simulink model "debugUDP"  (Simulink 7.2)
settings: Solver=ode1  SolverMode=SingleTasking  StartTime=0  StopTime=FAKEExpData.t(end)+4  FixedStep=0.001  RelTol=1e-3
PreLoadFcn:
  | InitModel
  | make
InitFcn:
  | InitModel
  | make
values from neighbouring files (symbols this model uses):
  D = SSD.D    [Ext_MPCPara.m]
  Ts = 0.002    [DSC_Control_Analysis.m]    (also in DSC_Control_Analysis_Exp.m; DSC_Speed_Control_Analysis.m; EC_params_nissan.m; Ext_MPCPara.m = SSD.Ts)
undefined symbols (not defined in the file or in its folder): FAKEExpData
libraries: xpclib x7, simulink x3
settings Model: Creator=cgadda  LastModifiedBy=ddl  ExtModeArmWhenConnect=off  ExtModeAutoUpdateStatusClock=off  BufferReuse=off
settings DataIOCC: LimitDataPoints=off  TimeSaveName=t  OutputSaveName=y  SignalLoggingName=sigsOut
settings OptimizationCC: BlockReduction=off  BooleanDataType=off  OptimizeBlockIOStorage=off  BufferReuse=off  EnforceIntegerDowncast=off  ExpressionFolding=off  FoldNonRolledExpr=off  LocalBlockOutputs=off  InitFltsAndDblsToZero=on
settings DebuggingCC: SaveWithParameterizedLinksMsg=none  SolverPrmCheckMsg=none  MultiTaskDSMMsg=warning  MultiTaskCondExecSysMsg=none
settings HardwareCC: ProdIntDivRoundTo=Zero  ProdEndianess=LittleEndian  ProdHWDeviceType=Generic->32-bit x86 compatible  TargetIntDivRoundTo=Zero  TargetEndianess=LittleEndian  TargetHWDeviceType=32-bit xPC Target (Intel Pentium)
settings RTWCC: SystemTargetFile=xpctarget.tlc  TemplateMakefile=xpc_default_tmf  Description=xPC Target  ProcessScript=xpctarget_make_rtw_hook  IncludeERTFirstTime=on  RTWCompilerOptimization=On
settings xpcTargetCC: TargetFcnLib=ansi_tfl_tmw.mat  TargetFunctionLibrary=ANSI_C  PortableWordSizes=off  RL32LogBufSizeModifier=25000000  xPCisDownloadable=off

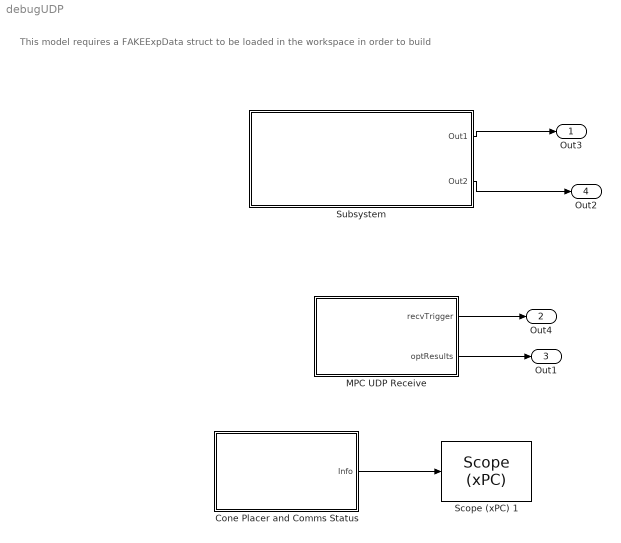
== system debugUDP ==
  note: This model requires a FAKEExpData struct
      | to be loaded in the workspace in order
      | to build
  Cone Placer and Comms Status : Subsystem
  MPC UDP Receive : Subsystem
  Scope (xPC) 1 : xpclib/Misc./Scope (xPC)   SystemSampleTime=-1  scopeno=1  scopetype=Target  autostart=on  viewmode=Numerical  formatstr="' Bumper E Pos [m]:    %4.2f, Bumper N Pos [m]:    %4.2f, Num Laptop Msgs: %5.0f, Num Veh Msgs:    %5.0f'"  grid=on  ylimits=[0,0]  nosamples=round(1/Ts)  noprepostsamples=0  interleave=1  triggermode=FreeRun  triggersignal=1  triggerlevel=0.0  triggerslope=Either  triggerscope=1  triggersample=0  filename=data.dat  mode=Lazy  writesize=512  autorestart=off
  Subsystem : Subsystem
  Out3 : Outport  OutDataType=sfix(16)  OutScaling=2^0
  Out4 : Outport  Port=2  OutDataType=sfix(16)  OutScaling=2^0
  Out1 : Outport  Port=3  OutDataType=sfix(16)  OutScaling=2^0
  Out2 : Outport  Port=4  OutDataType=sfix(16)  OutScaling=2^0
  wires:
  Subsystem/2(Out2) -> Out2/1
  MPC UDP Receive/2(optResults) -> Out1/1
  MPC UDP Receive/1(recvTrigger) -> Out4/1
  Subsystem/1(Out1) -> Out3/1
  Cone Placer and Comms Status/1(Info) -> Scope (xPC) 1/1

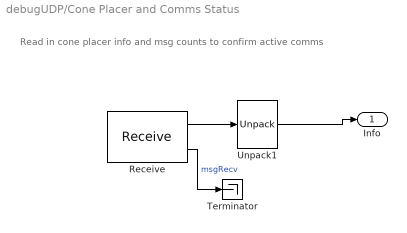
== system debugUDP/Cone Placer and Comms Status ==
  note: Read in cone
      | placer info and
      | msg counts to confirm
      | active comms
  Receive : xpclib/UDP/Receive  ipAddress=171.64.164.232  ipPort=25012  width=4*8  sampletime=-1
  Terminator : Terminator
  Unpack1 : xpclib/UDP/Unpack  dimensions={4}  datatypes={'double'}  byteAlign=1
  Info : Outport  OutDataType=sfix(16)  OutScaling=2^0
  wires:
  Receive/1 -> Unpack1/1
  Unpack1/1 -> Info/1
  Receive/2 -> Terminator/1  "msgRecv"

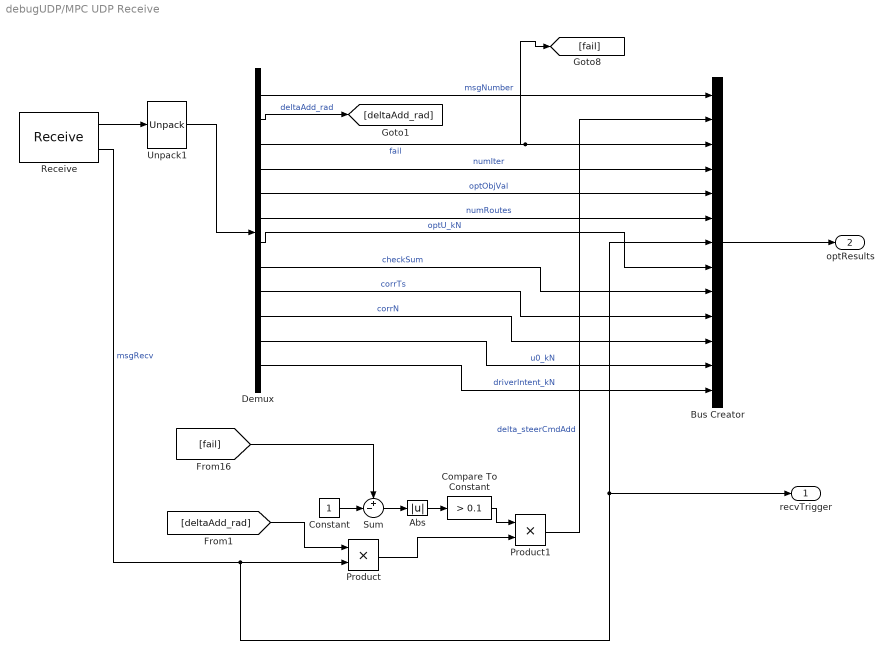
== system debugUDP/MPC UDP Receive ==
  Abs : Abs  OutDataType=sfix(16)  OutScaling=2^0
  Bus Creator : BusCreator  Inputs=13
  Compare To Constant : simulink/Logic and Bit Operations/Compare To Constant  SystemSampleTime=-1  relop=>  const=0.1  LogicOutDataTypeMode=uint8  ZeroCross=off
  Constant : Constant  OutDataType=sfix(16)  OutScaling=2^0
  Demux : Demux  Outputs=12
  Product : Product  OutDataType=sfix(16)  OutScaling=2^0  RndMeth=Zero
  Product1 : Product  OutDataType=sfix(16)  OutScaling=2^0  RndMeth=Zero
  Receive : xpclib/UDP/Receive  ipAddress=171.64.164.232  ipPort=25011  width=12*8  sampletime=-1
  Sum : Sum  Inputs=+-|  OutDataType=sfix(16)  OutScaling=2^0
  Unpack1 : xpclib/UDP/Unpack  dimensions={12}  datatypes={'double'}  byteAlign=1
  recvTrigger : Outport  OutDataType=sfix(16)  OutScaling=2^0
  optResults : Outport  Port=2  OutDataType=sfix(16)  OutScaling=2^0
  wires:
  Receive/1 -> Unpack1/1
  Receive/2 -> Product/2, Bus Creator/7, recvTrigger/1  "msgRecv"
  Unpack1/1 -> Demux/1
  Demux/1 -> Bus Creator/1  "msgNumber"
  Demux/3 -> Bus Creator/3, [fail]  "fail"
  Demux/4 -> Bus Creator/4  "numIter"
  Demux/5 -> Bus Creator/5  "optObjVal"
  Product1/1 -> Bus Creator/2  "delta_steerCmdAdd"
  Constant/1 -> Sum/2
  Sum/1 -> Abs/1
  Abs/1 -> Compare To Constant/1
  Compare To Constant/1 -> Product1/1
  Product/1 -> Product1/2
  Bus Creator/1 -> optResults/1
  Demux/7 -> Bus Creator/8  "optU_kN"
  Demux/8 -> Bus Creator/9  "checkSum"
  Demux/9 -> Bus Creator/10  "corrTs"
  Demux/10 -> Bus Creator/11  "corrN"
  Demux/11 -> Bus Creator/12  "u0_kN"
  Demux/12 -> Bus Creator/13  "driverIntent_kN"
  [fail] -> Sum/1
  Demux/2 -> [deltaAdd_rad]  "deltaAdd_rad"
  Demux/6 -> Bus Creator/6  "numRoutes"
  [deltaAdd_rad] -> Product/1

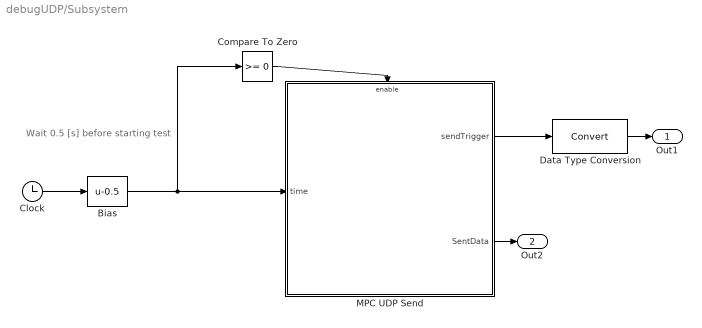
== system debugUDP/Subsystem ==
  note: Wait 0.5 [s] before
      | starting test
  Bias : Bias  Bias=-0.5
  Clock : Clock
      settings: Decimation=10
  Compare To Zero : simulink/Logic and Bit Operations/Compare To Zero  SystemSampleTime=-1  relop=>=  LogicOutDataTypeMode=uint8  ZeroCross=off
  Data Type Conversion : DataTypeConversion  OutDataType=sfix(16)  OutScaling=2^0
  MPC UDP Send : Subsystem
  Out1 : Outport
  Out2 : Outport  Port=2
  wires:
  MPC UDP Send/1(sendTrigger) -> Data Type Conversion/1
  Data Type Conversion/1 -> Out1/1
  MPC UDP Send/2(SentData) -> Out2/1
  Clock/1 -> Bias/1
  Bias/1 -> MPC UDP Send/1(time), Compare To Zero/1
  Compare To Zero/1 -> MPC UDP Send/Enable

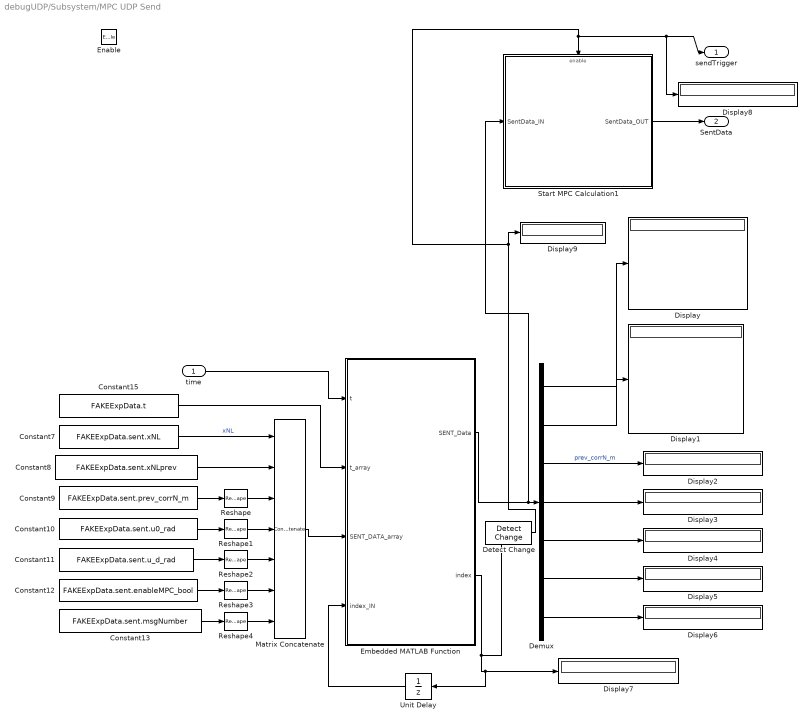
== system debugUDP/Subsystem/MPC UDP Send ==
  time : Inport  OutDataType=sfix(16)  OutScaling=2^0
  Enable : EnablePort
  Constant10 : Constant  Value=FAKEExpData.sent.u0_rad  OutDataType=sfix(16)  OutScaling=2^0
  Constant11 : Constant  Value=FAKEExpData.sent.u_d_rad  OutDataType=sfix(16)  OutScaling=2^0
  Constant12 : Constant  Value=FAKEExpData.sent.enableMPC_bool  OutDataType=sfix(16)  OutScaling=2^0
  Constant13 : Constant  Value=FAKEExpData.sent.msgNumber  OutDataType=sfix(16)  OutScaling=2^0
  Constant15 : Constant  Value=FAKEExpData.t  OutDataType=sfix(16)  OutScaling=2^0
  Constant7 : Constant  Value=FAKEExpData.sent.xNL  OutDataType=sfix(16)  OutScaling=2^0
  Constant8 : Constant  Value=FAKEExpData.sent.xNLprev  OutDataType=sfix(16)  OutScaling=2^0
  Constant9 : Constant  Value=FAKEExpData.sent.prev_corrN_m  OutDataType=sfix(16)  OutScaling=2^0
  Demux : Demux  Outputs=[6 6 1 1 1 1 1]
  Detect Change : simulink/Logic and Bit Operations/Detect Change  SystemSampleTime=-1  vinit=-1
  Display{,1..9} (10 alike) : Display
  Embedded MATLAB Function : Stateflow chart
  Matrix Concatenate : Concatenate  NumInputs=7  Mode=Multidimensional array
  Reshape{,1..4} (5 alike) : Reshape  OutputDimensionality=Row vector (2-D)
  Start MPC Calculation1 : Subsystem  TreatAsAtomicUnit=on
  Unit Delay : UnitDelay  Orientation=left  X0=1
  sendTrigger : Outport  OutDataType=sfix(16)  OutScaling=2^0
  SentData : Outport  Port=2  OutDataType=sfix(16)  OutScaling=2^0
  wires:
  Start MPC Calculation1/1(SentData_OUT) -> SentData/1
  time/1 -> Embedded MATLAB Function/1(t)
  Constant15/1 -> Embedded MATLAB Function/2(t_array)
  Constant7/1 -> Matrix Concatenate/1  "xNL"
  Constant8/1 -> Matrix Concatenate/2
  Constant9/1 -> Reshape/1
  Constant10/1 -> Reshape1/1
  Constant11/1 -> Reshape2/1
  Constant12/1 -> Reshape3/1
  Constant13/1 -> Reshape4/1
  Matrix Concatenate/1 -> Embedded MATLAB Function/3(SENT_DATA_array)
  Embedded MATLAB Function/1(SENT_Data) -> Demux/1, Start MPC Calculation1/1(SentData_IN)
  Reshape/1 -> Matrix Concatenate/3
  Reshape1/1 -> Matrix Concatenate/4
  Reshape2/1 -> Matrix Concatenate/5
  Reshape3/1 -> Matrix Concatenate/6
  Reshape4/1 -> Matrix Concatenate/7
  Demux/1 -> Display/1
  Demux/2 -> Display1/1
  Demux/3 -> Display2/1  "prev_corrN_m"
  Demux/4 -> Display3/1
  Demux/5 -> Display4/1
  Demux/6 -> Display5/1
  Demux/7 -> Display6/1
  Embedded MATLAB Function/2(index) -> Unit Delay/1, Display7/1, Detect Change/1
  Unit Delay/1 -> Embedded MATLAB Function/4(index_IN)
  Detect Change/1 -> Display9/1, Start MPC Calculation1/Enable, sendTrigger/1, Display8/1

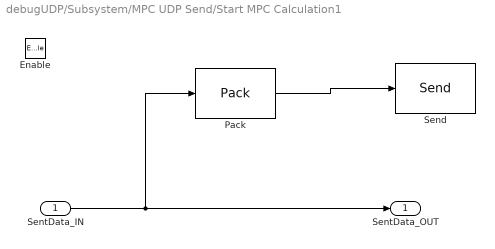
== system debugUDP/Subsystem/MPC UDP Send/Start MPC Calculation1 ==
  SentData_IN : Inport  OutDataType=sfix(16)  OutScaling=2^0
  Enable : EnablePort
  Pack : xpclib/UDP/Pack  datatypes={'double'}  byteAlign=1
  Send : xpclib/UDP/Send  ipAddress=171.64.164.232  ipPort=25001  localPort=25001  sampletime=-1
  SentData_OUT : Outport  OutDataType=sfix(16)  OutScaling=2^0
  wires:
  Pack/1 -> Send/1
  SentData_IN/1 -> Pack/1, SentData_OUT/1

== matlab function Subsystem/MPC UDP Send/Embedded MATLAB Function ==
  data: t input double; t_array input double; SENT_DATA_array input double; SENT_Data output double; index output double; index_IN input double
function [SENT_Data, index] = fcn(t, t_array, SENT_DATA_array, index_IN)
% This block supports the Embedded MATLAB subset.
% See the help menu for details. 
index = index_IN;

myEps = abs(index - length(t_array));

if (myEps < 1e-7)
    % do nothing, just hold last data
else
    %% find current time
    eps = abs(t-t_array(index));
    while (~(eps < 1e-7) && ~((t_array(index) < t) && (t_array(index+1) > t)))
        index = index+1;
        eps = abs(t-t_array(index));
        if (index == length(t_array))
            break;
        end
    end
end

SENT_Data = SENT_DATA_array(:,index);
